simulink subsystem "PieroModelS"  (R2023b)
settings: Solver=VariableStepAuto  StartTime=0.0  StopTime=10.0  RelTol=1e-3
settings Model: Creator=Usuario  LastModifiedBy=Daniel

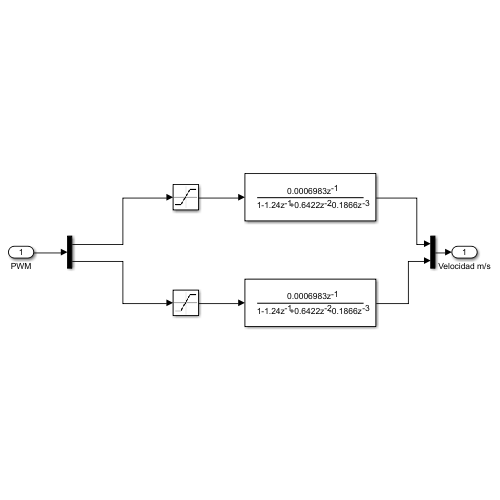
[thumbnail: Simulink's stored preview of the top-level diagram]
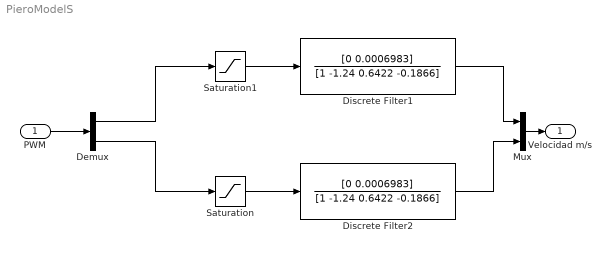
== system PieroModelS ==
  PWM : Inport
  Demux : Demux  Outputs=2
  Discrete Filter1 : DiscreteFilter  Numerator=[0 0.0006983]  Denominator=[1 -1.24 0.6422 -0.1866]
  Discrete Filter2 : DiscreteFilter  Numerator=[0 0.0006983]  Denominator=[1 -1.24 0.6422 -0.1866]
  Mux : Mux  Inputs=2
  Saturation : Saturate  UpperLimit=255  LowerLimit=-255
  Saturation1 : Saturate  UpperLimit=255  LowerLimit=-255
  Velocidad m/s : Outport
  wires:
  Discrete Filter1/1 -> Mux/1
  Discrete Filter2/1 -> Mux/2
  PWM/1 -> Demux/1
  Mux/1 -> Velocidad m/s/1
  Demux/1 -> Saturation1/1
  Demux/2 -> Saturation/1
  Saturation/1 -> Discrete Filter2/1
  Saturation1/1 -> Discrete Filter1/1
